simulink model "Cruise_Control_dsgn"  (R2021a)
settings: Solver=VariableStepAuto  StartTime=0.0  StopTime=200  RelTol=1e-3
InitFcn:
  | Cruise_Control_design
values from neighbouring files (symbols this model uses):
  Kd = 0    [Cruise_Control_design.m]
  Ki = 10.1187    [Cruise_Control_design.m]
  Kp = 174.6119    [Cruise_Control_design.m]
  m = 1084    [Cruise_Control_design.m]
  plant_den = [1 1/50.5355]    [Cruise_Control_design.m]
  plant_num = 9.22123*1e-4    (= 0.000922123)    [Cruise_Control_design.m]
  V_set_speed = str2double(answer)    [Cruise_Control_design.m]
libraries: pid_lib x1
settings Model: Creator=ChOm1  LastModifiedBy=User
settings SolverCC: AlgebraicLoopSolver=TrustRegion
settings DebuggingCC: SFMachineParentedDataDiag=warning

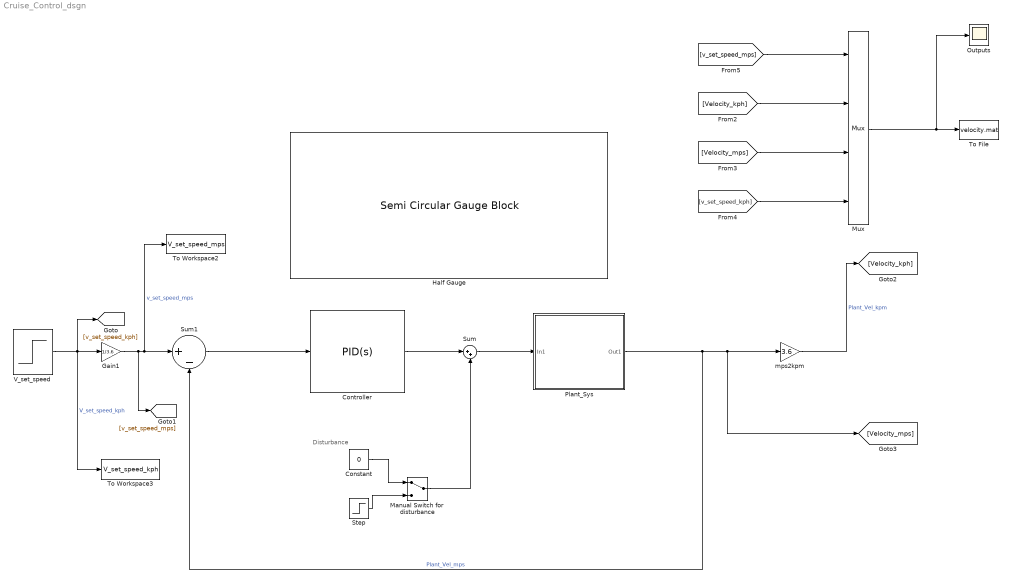
== system Cruise_Control_dsgn ==
  note: Disturbance
  Constant : Constant  Value=0
  Controller : pid_lib/PID Controller  Controller=PID  Form=Parallel  TimeDomain=Continuous-time  UseExternalTs=off  SampleTime=-1  IntegratorMethod=Forward Euler  FilterMethod=Forward Euler  ControllerParametersSource=internal  P=Kp  I=Ki  D=Kd  UseFilter=on  N=100  TunerSelectOption=Transfer Function Based (PID Tuner App)  InitialConditionSource=internal  InitialConditionForIntegrator=0  InitialConditionForFilter=0  DifferentiatorICPrevScaledInput=0  ExternalReset=none  TrackingMode=off  Kt=1  LimitOutput=off  SatLimitsSource=internal  UpperSaturationLimit=inf  LowerSaturationLimit=-inf  LinearizeAsGain=on  AntiWindupMode=none  Kb=1  POutMin=[]  POutMax=[]  IOutMin=[]  IOutMax=[]  DOutMin=[]  DOutMax=[]  NOutMin=[]  NOutMax=[]  SumOutMin=[]  SumOutMax=[]  SaturationOutMin=[]  SaturationOutMax=[]  PParamMin=[]  PParamMax=[]  IParamMin=[]  IParamMax=[]  DParamMin=[]  DParamMax=[]  NParamMin=[]  NParamMax=[]  KbParamMin=[]  KbParamMax=[]  KtParamMin=[]  KtParamMax=[]  KbOutMin=[]  KbOutMax=[]  KtOutMin=[]  KtOutMax=[]  IntegratorOutMin=[]  IntegratorOutMax=[]  FilterOutMin=[]  FilterOutMax=[]  SumI1OutMin=[]  SumI1OutMax=[]  SumI2OutMin=[]  SumI2OutMax=[]  SumI3OutMin=[]  SumI3OutMax=[]  SumI4OutMin=[]  SumI4OutMax=[]  SumDOutMin=[]  SumDOutMax=[]  DifferentiatorOutMin=[]  DifferentiatorOutMax=[]  FilterDiffOutCoefMin=[]  FilterDiffOutCoefMax=[]  ReciprocalOutMin=[]  ReciprocalOutMax=[]  SumDenOutMin=[]  SumDenOutMax=[]  SumNumOutMin=[]  SumNumOutMax=[]  DivideOutMin=[]  DivideOutMax=[]  UdiffTsProdOutMin=[]  UdiffTsProdOutMax=[]  NTsProdOutMin=[]  NTsProdOutMax=[]  UintegralTsProdOutMin=[]  UintegralTsProdOutMax=[]  UngainTsProdOutMin=[]  UngainTsProdOutMax=[]  IntegratorContinuousStateAttributes=''  IntegratorStateMustResolveToSignalObject=off  IntegratorRTWStateStorageClass=Auto  FilterContinuousStateAttributes=''  FilterStateMustResolveToSignalObject=off  FilterRTWStateStorageClass=Auto  ParallelPVariant=InternalParameters  IdealPVariant=Disabled  IVariant=InternalParameters  DVariant=InternalParameters  IntegratorVariant=Continuous  SatVariant=Disabled  AWVariant=Passthrough  PCopyVariant=Disabled  TRVariant=Disabled  FdbkBlocksVariant=Forward  IdealPFdbkVariant=Disabled  SatFdbkVariant=Disabled  DerivativeFilterVariant=ContFilter  NVariant=InternalParameters  NCopyVariant=Disabled  FilterICVariant=InternalICsFilter  IntegratorICVariant=InternalICs  ExternalResetVariant=Disabled  TRSumVariant=Passthrough  SumFdbkVariant=Disabled  SumVariant=Sum_PID  TsampFilterVariant=InternalTs  TsampNgainVariant=Passthrough  TsampIntegralVariant=Passthrough  ExternalSaturationOutDataTypeStr=Inherit: Same as second input
  Gain1 : Gain  Gain=1/3.6
  Half Gauge : SemiCircularGaugeBlock  ScaleMax=250
  Manual Switch for  disturbance : ManualSwitch
  Mux : Mux
  Outputs : Scope
  Plant_Sys : Subsystem
  Step : Step  Time=100  After=m*9.81*sin(pi/45)  SampleTime=0
  Sum : Sum  Inputs=|++
  Sum1 : Sum  Inputs=|+-
  To File : ToFile  Filename=velocity.mat
  To Workspace2 : ToWorkspace  VariableName=V_set_speed_mps  SaveFormat=Timeseries  SampleTime=-1
  To Workspace3 : ToWorkspace  VariableName=V_set_speed_kph  SaveFormat=Timeseries  SampleTime=-1
  V_set_speed : Step  After=V_set_speed  SampleTime=0
  mps2kpm : Gain  Gain=3.6
  wires:
  mps2kpm/1 -> [Velocity_kph]  "Plant_Vel_kpm"
  Plant_Sys/1(Out1) -> Sum1/2, [Velocity_mps], mps2kpm/1  "Plant_Vel_mps"
  Controller/1 -> Sum/1
  Sum/1 -> Plant_Sys/1(In1)
  Constant/1 -> Manual Switch for  disturbance/1
  Step/1 -> Manual Switch for  disturbance/2
  Manual Switch for  disturbance/1 -> Sum/2
  Sum1/1 -> Controller/1
  V_set_speed/1 -> To Workspace3/1, [v_set_speed_kph], Gain1/1  "V_set_speed_kph"
  Gain1/1 -> Sum1/1, To Workspace2/1, [v_set_speed_mps]  "v_set_speed_mps"
  [v_set_speed_kph] -> Mux/4
  [Velocity_mps] -> Mux/3
  [Velocity_kph] -> Mux/2
  [v_set_speed_mps] -> Mux/1
  Mux/1 -> Outputs/1, To File/1

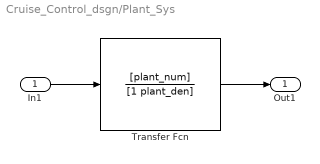
== system Cruise_Control_dsgn/Plant_Sys ==
  In1 : Inport
  Transfer Fcn : TransferFcn  Numerator=[plant_num]  Denominator=[1 plant_den]
  Out1 : Outport
  wires:
  In1/1 -> Transfer Fcn/1
  Transfer Fcn/1 -> Out1/1
